simulink subsystem "anode_subsystem_controller"  (R2023a)
settings: Solver=VariableStepAuto  StartTime=0.0  StopTime=10.0  RelTol=1e-3
values from neighbouring files (symbols this model uses):
  densityHydrogen = 0.0899    [All_Properties.mat]    (also in Valve_Init.m; anode_subsystem_parameters.m)
  Kv_VL6112 = 0.8    [All_Properties.mat]    (also in anode_subsystem_parameters.m)
libraries: nesl_utility x5, fl_lib x4
settings Model: Creator=stefan.notter  LastModifiedBy=debjani.ghosh

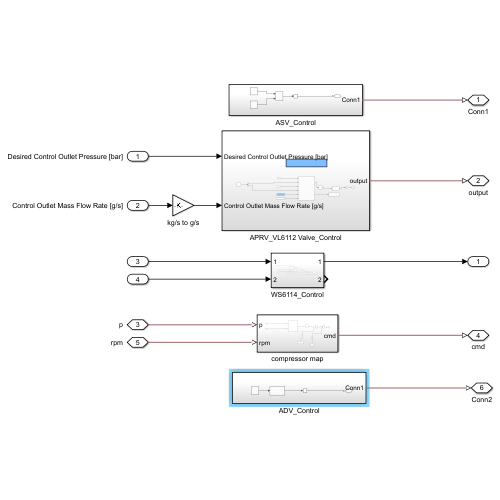
[thumbnail: Simulink's stored preview of the top-level diagram]
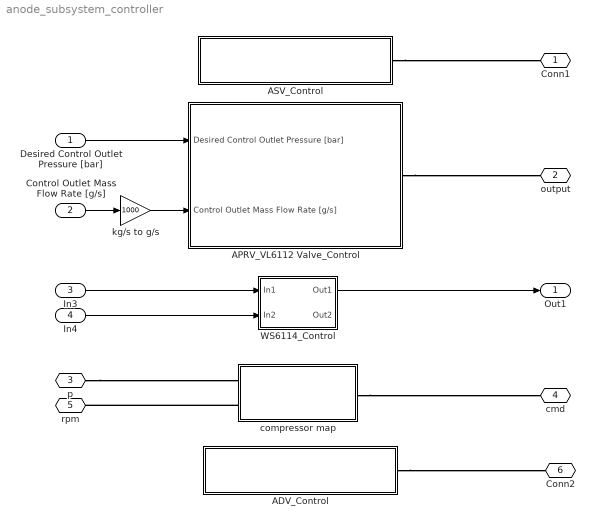
== system anode_subsystem_controller ==
  Desired Control Outlet Pressure [bar] : Inport
  Control Outlet Mass Flow Rate [g/s] : Inport  Port=2
  In3 : Inport  Port=3
  In4 : Inport  Port=4
  ADV_Control : Subsystem
  APRV_VL6112 Valve_Control : Subsystem
  ASV_Control : Subsystem
  WS6114_Control : Subsystem
  compressor map : Subsystem
  kg/s to g/s : Gain  Gain=1000
  Conn1 : PMIOPort  Side=Right
  output : PMIOPort  Port=2  Side=Right
  p : PMIOPort  Port=3  Side=Left
  cmd : PMIOPort  Port=4  Side=Right
  rpm : PMIOPort  Port=5  Side=Left
  Conn2 : PMIOPort  Port=6  Side=Right
  Out1 : Outport
  wires:
  Control Outlet Mass Flow Rate [g/s]/1 -> kg/s to g/s/1
  WS6114_Control/1(Out1) -> Out1/1
  In3/1 -> WS6114_Control/1(In1)
  In4/1 -> WS6114_Control/2(In2)
  kg/s to g/s/1 -> APRV_VL6112 Valve_Control/2(Control Outlet Mass Flow Rate [g/s])
  Desired Control Outlet Pressure [bar]/1 -> APRV_VL6112 Valve_Control/1(Desired Control Outlet Pressure [bar])
  connections:
  p/RConn1 -- compressor map/LConn1
  ASV_Control/RConn1 -- Conn1/RConn1
  compressor map/RConn1 -- cmd/RConn1
  compressor map/LConn2 -- rpm/RConn1
  APRV_VL6112 Valve_Control/RConn1 -- output/RConn1
  ADV_Control/RConn1 -- Conn2/RConn1

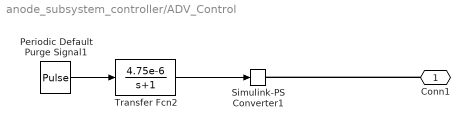
== system anode_subsystem_controller/ADV_Control ==
  Periodic Default Purge Signal1 : DiscretePulseGenerator  PulseType=Time based  Period=3  PulseWidth=5
  Simulink-PS Converter1 : nesl_utility/Simulink-PS Converter  PhysicalDomain=network_engine_domain  SubClassName=ps_input  LeftPortType=input  RightPortType=output  PseudoPeriodic=off  Frequencies=[]  NoiseDistribution=none  NoiseParameters=[]  Unit=m^2  AffineConversion=off  FilteringAndDerivatives=provide  SimscapeFilterOrder=1  InputFilterTimeConstant=0.001  UdotUserProvided=0
  Transfer Fcn2 : TransferFcn  Numerator=[4.75e-6]  Denominator=[1 1]
  Conn1 : PMIOPort  Side=Right
  wires:
  Transfer Fcn2/1 -> Simulink-PS Converter1/1
  Periodic Default Purge Signal1/1 -> Transfer Fcn2/1
  connections:
  Conn1/RConn1 -- Simulink-PS Converter1/RConn1

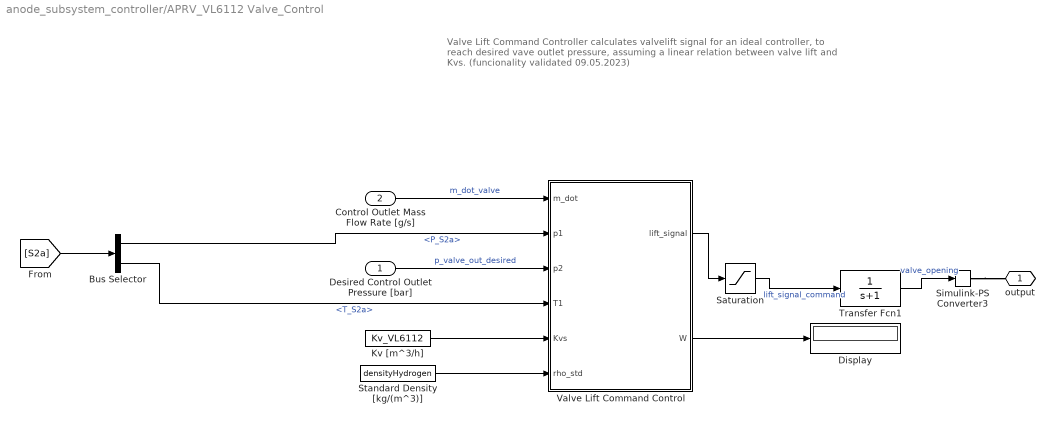
== system anode_subsystem_controller/APRV_VL6112 Valve_Control ==
  note: Valve Lift Command Controller calculates valvelift signal for an
      | ideal controller, to reach desired vave outlet pressure, assuming
      | a linear relation between valve lift and Kvs.
      | (funcionality validated 09.05.2023)
  Desired Control Outlet Pressure [bar] : Inport
  Control Outlet Mass Flow Rate [g/s] : Inport  Port=2
  Bus Selector : BusSelector  OutputSignals=P_S2a,T_S2a
  Display : Display
  Kv [m^3/h] : Constant  Value=Kv_VL6112
  Saturation : Saturate  UpperLimit=1  LowerLimit=0
  Simulink-PS Converter3 : nesl_utility/Simulink-PS Converter  PhysicalDomain=network_engine_domain  SubClassName=ps_input  LeftPortType=input  RightPortType=output  PseudoPeriodic=off  Frequencies=[]  NoiseDistribution=none  NoiseParameters=[]  Unit=m^2  AffineConversion=off  FilteringAndDerivatives=provide  SimscapeFilterOrder=1  InputFilterTimeConstant=0.001  UdotUserProvided=0
  Standard Density [kg/(m^3)] : Constant  Value=densityHydrogen
  Transfer Fcn1 : TransferFcn  Denominator=[1 1]
  Valve Lift Command Control : MATLAB Function  TreatAsAtomicUnit=on
  output : PMIOPort  Side=Right
  wires:
  Desired Control Outlet Pressure [bar]/1 -> Valve Lift Command Control/3(p2)  "p_valve_out_desired"
  Valve Lift Command Control/1(lift_signal) -> Saturation/1
  Kv [m^3/h]/1 -> Valve Lift Command Control/5(Kvs)
  [S2a] -> Bus Selector/1
  Control Outlet Mass Flow Rate [g/s]/1 -> Valve Lift Command Control/1(m_dot)  "m_dot_valve"
  Bus Selector/2 -> Valve Lift Command Control/4(T1)  "<T_S2a>"
  Saturation/1 -> Transfer Fcn1/1  "lift_signal_command"
  Standard Density [kg/(m^3)]/1 -> Valve Lift Command Control/6(rho_std)
  Transfer Fcn1/1 -> Simulink-PS Converter3/1  "valve_opening"
  Valve Lift Command Control/2(W) -> Display/1
  Bus Selector/1 -> Valve Lift Command Control/2(p1)  "<P_S2a>"
  connections:
  Simulink-PS Converter3/RConn1 -- output/RConn1

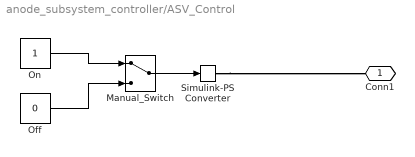
== system anode_subsystem_controller/ASV_Control ==
  Manual_Switch : ManualSwitch
  Off : Constant  Value=0
  On : Constant
  Simulink-PS Converter : nesl_utility/Simulink-PS Converter  PhysicalDomain=network_engine_domain  SubClassName=ps_input  LeftPortType=input  RightPortType=output  PseudoPeriodic=off  Frequencies=[]  NoiseDistribution=none  NoiseParameters=[]  Unit=1  AffineConversion=off  FilteringAndDerivatives=provide  SimscapeFilterOrder=1  InputFilterTimeConstant=0.001  UdotUserProvided=0
  Conn1 : PMIOPort  Side=Right
  wires:
  Off/1 -> Manual_Switch/2
  On/1 -> Manual_Switch/1
  Manual_Switch/1 -> Simulink-PS Converter/1
  connections:
  Simulink-PS Converter/RConn1 -- Conn1/RConn1

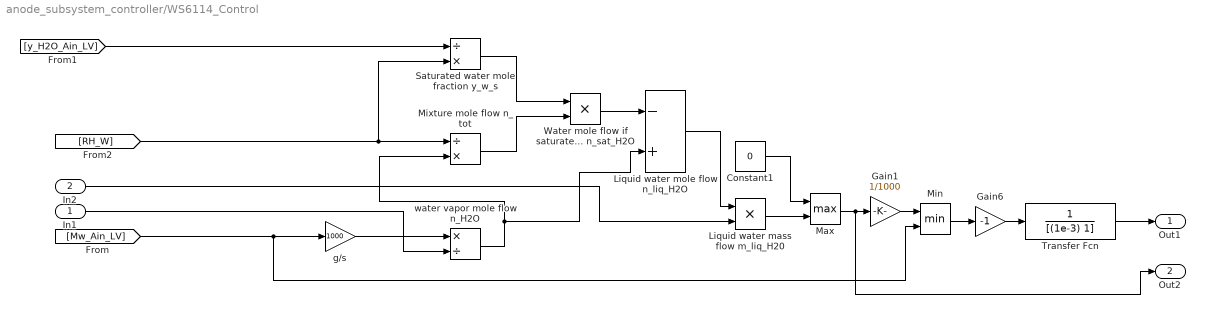
== system anode_subsystem_controller/WS6114_Control ==
  In1 : Inport
  In2 : Inport  Port=2
  Constant1 : Constant  Value=0
  Gain1 : Gain  Gain=1/1000
  Gain6 : Gain  Gain=-1
  Liquid water mass flow m_liq_H20 : Product
  Liquid water mole flow n_liq_H2O : Sum  Inputs=-+
  Max : MinMax  Function=max  Inputs=2
  Min : MinMax  Inputs=2
  Mixture mole flow n_tot : Product  Inputs=/*
  Saturated water mole fraction y_w_s : Product  Inputs=/*
  Transfer Fcn : TransferFcn  Denominator=[(1e-3) 1]
  Water mole flow if saturated n_sat_H2O : Product
  g/s : Gain  Gain=1000
  water vapor mole flow n_H2O : Product  Inputs=*/
  Out1 : Outport
  Out2 : Outport  Port=2
  wires:
  Saturated water mole fraction y_w_s/1 -> Water mole flow if saturated n_sat_H2O/1
  [y_H2O_Ain_LV] -> Saturated water mole fraction y_w_s/1
  Transfer Fcn/1 -> Out1/1
  [RH_W] -> Saturated water mole fraction y_w_s/2, Mixture mole flow n_tot/1
  Water mole flow if saturated n_sat_H2O/1 -> Liquid water mole flow n_liq_H2O/1
  Liquid water mass flow m_liq_H20/1 -> Max/2
  Mixture mole flow n_tot/1 -> Water mole flow if saturated n_sat_H2O/2
  Gain6/1 -> Transfer Fcn/1
  Gain1/1 -> Min/1
  In2/1 -> Liquid water mass flow m_liq_H20/2
  Liquid water mole flow n_liq_H2O/1 -> Liquid water mass flow m_liq_H20/1
  g/s/1 -> water vapor mole flow n_H2O/1
  In1/1 -> water vapor mole flow n_H2O/2
  Constant1/1 -> Max/1
  Min/1 -> Gain6/1
  water vapor mole flow n_H2O/1 -> Liquid water mole flow n_liq_H2O/2, Mixture mole flow n_tot/2
  [Mw_Ain_LV] -> g/s/1, Min/2
  Max/1 -> Out2/1, Gain1/1

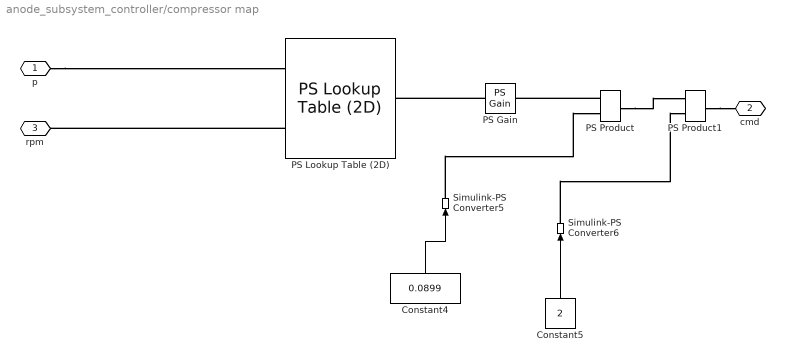
== system anode_subsystem_controller/compressor map ==
  Constant4 : Constant  Value=0.0899
  Constant5 : Constant  Value=2
  PS Gain : fl_lib/Physical Signals/Functions/PS Gain  gain=1/3600
  PS Lookup Table (2D) : fl_lib/Physical Signals/Lookup Tables/PS Lookup Table (2D)  x1=comp6122_p_out  x2=comp6122_rpm  f=comp6122_V_dot  interp_method=simscape.enum.interpolation.linear  extrap_method=simscape.enum.extrapolation.linear
  PS Product : fl_lib/Physical Signals/Functions/PS Product
  PS Product1 : fl_lib/Physical Signals/Functions/PS Product
  Simulink-PS Converter5 : nesl_utility/Simulink-PS Converter  PhysicalDomain=network_engine_domain  SubClassName=ps_input  LeftPortType=input  RightPortType=output  PseudoPeriodic=off  Frequencies=[]  NoiseDistribution=none  NoiseParameters=[]  Unit=1  AffineConversion=on  FilteringAndDerivatives=provide  SimscapeFilterOrder=1  InputFilterTimeConstant=0.001  UdotUserProvided=0
  Simulink-PS Converter6 : nesl_utility/Simulink-PS Converter  PhysicalDomain=network_engine_domain  SubClassName=ps_input  LeftPortType=input  RightPortType=output  PseudoPeriodic=off  Frequencies=[]  NoiseDistribution=none  NoiseParameters=[]  Unit=1  AffineConversion=on  FilteringAndDerivatives=provide  SimscapeFilterOrder=1  InputFilterTimeConstant=0.001  UdotUserProvided=0
  p : PMIOPort  Side=Left
  cmd : PMIOPort  Port=2  Side=Right
  rpm : PMIOPort  Port=3  Side=Left
  wires:
  Constant5/1 -> Simulink-PS Converter6/1
  Constant4/1 -> Simulink-PS Converter5/1
  connections:
  p/RConn1 -- PS Lookup Table (2D)/LConn1
  PS Product1/RConn1 -- cmd/RConn1
  Simulink-PS Converter6/RConn1 -- PS Product1/LConn2
  PS Lookup Table (2D)/LConn2 -- rpm/RConn1
  PS Product/LConn1 -- PS Gain/RConn1
  PS Product/RConn1 -- PS Product1/LConn1
  PS Gain/LConn1 -- PS Lookup Table (2D)/RConn1
  Simulink-PS Converter5/RConn1 -- PS Product/LConn2

== matlab function anode_subsystem_controller/APRV_VL6112 Valve_Control/Valve Lift Command Control ==
  data: m_dot input; p1 input; p2 input; T1 input; Kvs input; lift_signal output; rho_std input; W output
function [lift_signal,W]  = fcn(m_dot,p1,p2,T1,Kvs,rho_std)

% calculation based on Bürkert. Direktwirkendes 2-Wege-Standard-Proportionalventil. Datenblatt
% for calculation based on Swagelok. Valve Sizing. Technical Bulletin:
% check calculation_valve_formulas_comparison

% determine optimum valve opening based on pressure ratio for subscritical conditions
% Kvs - valve coefficient [m^3/h] at fully valve open
% lift_signal = Kv/Kvs (linear assumption)

dp = max(0,p1 - p2);            % avoid complex square root

% distinction of flow characteristics based on pressure drop
if p2/p1 > 0.5
    % low pressure drop - subsonic flow
    lift_signal = m_dot*3.6/(Kvs*514)*sqrt(T1/(p2*dp*rho_std));
    W=1;
  
else 
    % high pressure drop - sonic flow (independent of downstream pressure)
    %lift_signal = 0.05;
    lift_signal = m_dot*3.6/(Kvs*257*p1)*sqrt(T1/rho_std);
     W=2;
end
